simulink model "verify"  (R2018b)
settings: Solver=ode14x  StartTime=0.0  StopTime=10.0  FixedStep=0.01  RelTol=1e-3
values from neighbouring files (symbols this model uses):
  cd = kp+kd*dfod*s    [phiz_cal15.m]
settings Model: Creator=lenovo  LastModifiedBy=standard
settings SFSimCC: SimUseLocalCustomCode=off
settings RTWCC: RTWUseLocalCustomCode=off

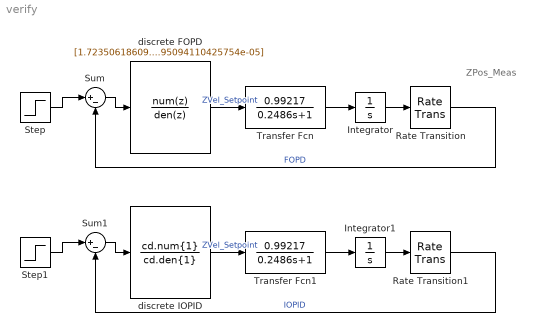
== system verify ==
  note: ZPos_Meas
  Integrator : Integrator
  Integrator1 : Integrator
  Rate Transition : RateTransition  OutPortSampleTime=0.01
  Rate Transition1 : RateTransition  OutPortSampleTime=0.01
  Step : Step  SampleTime=0.01
  Step1 : Step  SampleTime=0.01
  Sum : Sum  Inputs=|+-
  Sum1 : Sum  Inputs=|+-
  Transfer Fcn : TransferFcn  Numerator=[0.99217]  Denominator=[0.2486 1]
  Transfer Fcn1 : TransferFcn  Numerator=[0.99217]  Denominator=[0.2486 1]
  discrete FOPD : DiscreteTransferFcn  Numerator=[1.72350618609064,-5.70339892298403,7.11891293410561,-4.08227197470563,1.02223847578118,-0.0786444191365231]  Denominator=[0.0101201839324044,-0.0228427827690589,0.0162967440497079,-0.00320636053105791,-0.000423005899049262,8.95094110425754e-05]  SampleTime=0.01
  discrete IOPID : DiscreteTransferFcn  Numerator=cd.num{1}  Denominator=cd.den{1}  SampleTime=0.01
  wires:
  Step/1 -> Sum/1
  Sum/1 -> discrete FOPD/1
  discrete FOPD/1 -> Transfer Fcn/1  "ZVel_Setpoint"
  Transfer Fcn/1 -> Integrator/1
  Integrator/1 -> Rate Transition/1
  Rate Transition/1 -> Sum/2  "FOPD"
  Step1/1 -> Sum1/1
  discrete IOPID/1 -> Transfer Fcn1/1  "ZVel_Setpoint"
  Sum1/1 -> discrete IOPID/1
  Transfer Fcn1/1 -> Integrator1/1
  Rate Transition1/1 -> Sum1/2  "IOPID"
  Integrator1/1 -> Rate Transition1/1
